simulink model "Transicao"  (R2015b)
settings: Solver=FixedStepAuto  StartTime=0  StopTime=120  FixedStep=sampleTime  RelTol=1e-3
InitFcn:
  | sampleTime = 0.01;
  | Ktd = 0.0526/1000;
  | Kdd = 0.0526/1000;
  | Lb = [0.27 0.27 0.27 0.27];
  | LbAssimetrico  = [0.27 0.27 0.18 0.36];
  | LbTeste  = [0.27 0.27 0.18 0.36];
  | Ixx = 0.0754483;
  | Iyy = 0.13642;
  | Izz = 0.2043333;
  | 
  | IXYZ = [Ixx 0 0; 0 Iyy 0; 0 0 Izz];
  | 
  | areaLateral = [0.0114398 0 0; 0 0.09533687 0; 0 0 0.33];
  | 
  | areaAsa = 0.243;
  | areaProfundor = 0.051;
  | densidadeAr = 1.2;
  | cdArrastoParasita = 1.5;
  | clAviao = 0.825;
  | cdAviao = 0.0743;
  | g = 9.8;
  | massa = 3;
  | velCruzeiro = 15;
  | 
  | inicioTransicao = 40;
  | inicioDesativaAtivacao = 80;
  | 
  | global kroll
  | global kpitch
  | global kyaw
  | 
  | global kx
  | global ky
  | global kz
  | 
  | %Voo em cruzeiro
  | global ku
  | global kzprof
  | global kpitchprof
undefined symbols (not defined in the file or in its folder): DiscIntNeverNeededParam, kpitch, kpitchprof, kroll, ku, kx, kyaw, kz, kzprof
libraries: simulink x17, aerolibwind2 x1
(part 2 of 2)

== matlab function Transicao/Dinâmica do sistema/Dinâmica do sistema ==
  data: w1 input; w2 input; w3 input; w4 input; estados output; gravidade input; massaTotal input; rho input; areaAviao input; areaAsa input; cdParasita input; cdAviao input; clAviao input; ktd input; kdd input; lb input; Ixyz input; velVento input; beta input; alphaProfundor input; dt input; estados_anterior input; U output; a_angular output; a output; XYZ output; XYZ_ponto output; XYZ_ponto_ponto output; phi_theta_psi output; phi_theta_psi_ponto output; thrustX output; arrastoParasita output; arrastoInduzido output; sustentacao output; arrastoTotal output; forcas output; gravidadeVec output
function [estados, U, a_angular, a, XYZ, XYZ_ponto,XYZ_ponto_ponto, phi_theta_psi, phi_theta_psi_ponto, thrustX, arrastoParasita, arrastoInduzido, sustentacao, arrastoTotal, forcas, gravidadeVec]  = fcn(w1,w2, w3, w4, gravidade, massaTotal,rho,areaAviao, areaAsa, cdParasita, cdAviao, clAviao, ktd, kdd, lb, Ixyz, velVento, beta, alphaProfundor, dt, estados_anterior)

XYZ = estados_anterior(:, 1);
XYZ_ponto = estados_anterior(:, 2);
phi_theta_psi = estados_anterior(:, 3);
phi_theta_psi_ponto = estados_anterior(:, 4);

roll = phi_theta_psi(1);
pitch = phi_theta_psi(2);
yaw = phi_theta_psi(3);

% for i = 1:numel(phi_theta_psi_ponto);
%    if(abs(phi_theta_psi_ponto(i)) < 10e-8)
%       phi_theta_psi_ponto(i) = 0;
%    end
%    
% end
% 
% % for i = 1:numel(theta_phi_psi);
% %    if(abs(theta_phi_psi(i)) < 10e-6)
% %       theta_phi_psi(i) = 0;
% %    end
% % end
% 
% for i = 1:numel(XYZ_ponto);
%    if(abs(XYZ_ponto(i)) < 10e-8)
%       XYZ_ponto(i) = 0;
%    end
% end

phi = roll;
theta = pitch;
psi = yaw;
% Matriz de rotação ZYX 
%matrizRotacao =     [cos(pitch)*cos(yaw) sin(roll)*sin(pitch)*cos(yaw)-cos(roll)*sin(yaw) cos(roll)*sin(pitch)*cos(yaw)+sin(roll)*sin(yaw);
%   cos(pitch)*sin(yaw) sin(roll)*sin(pitch)*sin(yaw)+cos(roll)*cos(yaw) cos(roll)*sin(pitch)*sin(yaw)-sin(roll)*cos(yaw);
%   -sin(pitch) sin(roll)*cos(pitch) cos(roll)*cos(pitch)];

%matrizRotacao =     [cos(phi)*cos(psi)-cos(theta)*sin(phi)*sin(psi) -cos(psi)*sin(phi)-cos(phi)*cos(theta)*sin(psi) sin(theta)*sin(psi) ;
%                     cos(theta)*cos(psi)*sin(phi)+cos(phi)*sin(psi) cos(phi)*cos(theta)*cos(psi)-sin(phi)*sin(psi) -cos(psi)*sin(theta) ;
%                     sin(phi)*sin(theta) cos(phi)*sin(theta) cos(theta)];

matrizRotacao =     [cos(theta)*cos(psi) cos(psi)*sin(theta)*sin(phi)-sin(psi)*cos(phi) cos(psi)*sin(theta)*cos(phi)+sin(psi)*sin(phi);
                     sin(psi)*cos(theta) sin(psi)*sin(theta)*sin(phi)+cos(psi)*cos(phi) sin(psi)*sin(theta)*cos(phi)-cos(psi)*sin(phi);
                     -sin(theta) cos(theta)*sin(phi) cos(theta)*cos(phi)];



%T = [1 sin(roll)*tan(pitch) cos(roll)*tan(pitch);
%    0 cos(roll) -sin(roll);
%    0 sin(roll)/cos(pitch) cos(roll)/cos(pitch)];

T = [1 0 -sin(theta);
    0 cos(phi) cos(theta)*sin(phi);
    0 -sin(phi) cos(theta)*cos(phi)];

% Encontra velocidades lineares e angulares no eixo do corpo com base no
% eixo inercial
vel_angular_body = T*phi_theta_psi_ponto;
vel_linear_body = matrizRotacao'*XYZ_ponto;

%Velocidade do vento no referencial do corpo
vel_vento_body = matrizRotacao'*velVento;

% Velocidade do corpo em relação ao vento
vel_aerodinamica_body = vel_linear_body-vel_vento_body;

w2ParaU = [ ktd      ktd     ktd      ktd;
           -ktd*lb(2)      ktd*lb(1)     ktd*lb(1)     -ktd*lb(2);
            ktd*lb(3)     -ktd*lb(4)     ktd*lb(3)     -ktd*lb(4);
           -kdd     -kdd       kdd      kdd];


       
U = w2ParaU * [w1^2*cos(beta); w2^2; w3^2*cos(beta); w4^2]; % Componente vertical, motor 1 e 3 estão em tilt com ângulo Beta
thrustX = [([ ktd      ktd     ktd      ktd]*[w1^2*sin(beta); 0; w3^2*sin(beta); 0]) ; 0 ; 0];% Componente da força horizontal, com motor tiltado

% Forças presentes no body frame axis
thrust = U(1)*[0; 0; 1];
forcas = -thrust;
arrastoParasita = -sign(vel_aerodinamica_body).*((rho*(vel_aerodinamica_body.^2)'*cdParasita*areaAviao/2)'); % Calcula arrasto parasita

if(vel_aerodinamica_body(1) > 0)
    arrastoInduzido = [-rho*vel_aerodinamica_body(1)^2*cdAviao*areaAsa/2 ; 0 ; 0]; % Encontra arrasto induzido da asa + profundor (o cd ta ajustado pra usar apenas a área da asa)
    clAlpha = 0.0744*(theta*180/pi +6) + 0.148;
    sustentacao = [0 ; 0 ; -rho*vel_aerodinamica_body(1)^2*clAlpha*areaAsa/2];
else
     arrastoInduzido = [0;0;0];
     sustentacao = [0;0;0];
end
arrastoTotal = arrastoParasita+arrastoInduzido;
gravidadeVec = (matrizRotacao')*(massaTotal*gravidade*[0; 0; 1]);
FtotalBody = -thrust + gravidadeVec + arrastoParasita+arrastoInduzido+sustentacao + thrustX; 

% Momentos presentes no body frame axis
mXroll = U(2);
mYpitch = U(3)+alphaProfundor;
mZyaw = U(4);
momentos = [mXroll; mYpitch; mZyaw];

% Adiciona efeito giroscópio e efeitos do produto vetorial do modelo de
% Newton-Euler
FtotalBody = FtotalBody - cross(vel_angular_body,(massaTotal*vel_linear_body));
momentos = momentos - cross(vel_angular_body,(Ixyz*vel_angular_body));

% Calcula aceleração em relação ao body frame
a = FtotalBody/massaTotal;

%Calcula aceleração angular em relação ao body frame
a_angular = inv(Ixyz)*(momentos);
%a_angular = inv(Ixyz)*(momentos);

% Resolvendo as tretas dos ângulos 
% https://i.imgur.com/82268P1.png
% Fonte: modelagem tese irada maluca

% Calcula velocidade angular em relação ao body axis
vel_angular_body = vel_angular_body + a_angular*dt;

% Encontra velocidade angular em relação ao eixo inercial
phi_theta_psi_ponto = inv(T)*vel_angular_body;

% Encontra os ângulos com base na velocidade angular no eixo inercial
phi_theta_psi = phi_theta_psi+ phi_theta_psi_ponto*dt;

% Encontra velocidade linear em relação ao body axis
vel_linear_body = vel_linear_body + a*dt;

XYZ_ponto_ponto = matrizRotacao*a;

% Encontra velocidade linear em relação ao eixo inercial
XYZ_ponto = matrizRotacao*vel_linear_body;

% Encontra posição em relação ao eixo inercial
XYZ = XYZ+XYZ_ponto*dt;

% if(modoCruzeiro == 1)
%     phi_theta_psi(2) = 0;
%     phi_theta_psi_ponto(2) = 0;
% end

estados = horzcat(XYZ, XYZ_ponto, phi_theta_psi, phi_theta_psi_ponto);

== matlab function Transicao/Atuador VTOL/Motor mixer ==
  data: u1thrust input; w1 output; u2mRoll input; u3mPitch input; u4mYaw input; w2 output; w3 output; w4 output; ktd input; kdd input; lb input
% Transforma um comando de thrust e momento em velocidade angular
function [w1,w2,w3,w4]= fcn(u1thrust, u2mRoll, u3mPitch, u4mYaw, ktd, kdd, lb)
% Supondo que U seja força e momentos
%w2ParaU = [ Ktd      Ktd     Ktd      Ktd;
%          -Ktd*Lb   Ktd*Lb  Ktd*Lb  -Ktd*Lb;
%           Ktd*Lb  -Ktd*Lb  Ktd*Lb  -Ktd*Lb;
%          -Kdd     -Kdd     Kdd      Kdd]

w2ParaU = [ ktd      ktd     ktd      ktd;
           -ktd*lb(2)      ktd*lb(1)     ktd*lb(1)     -ktd*lb(2);
            ktd*lb(3)     -ktd*lb(4)     ktd*lb(3)     -ktd*lb(4);
           -kdd     -kdd       kdd      kdd];


w = inv(w2ParaU)*[u1thrust ; u2mRoll ; u3mPitch ; u4mYaw];
for i = 1:numel(w);
   if(w(i) > 837.75^2)
      w(i) = 837.75^2; 
   end
end
for i = 1:numel(w);
   if(w(i) < 0)
      w(i) = 0; 
   end
end

w1 = sqrt(w(1));
w2 = sqrt(w(2));
w3 = sqrt(w(3));
w4 = sqrt(w(4));

== matlab function Transicao/Controle ângulo tilt/Controle Gain Schedualing ==
  data: velocidadeInercial input; phi_theta_psi input; betaFixo input; velAngularBeta input; tempoAtivacao input; sampleTime input; tempoSim input; betaAnterior input; beta output; velCruzeiro input; velCorpo output; modoAsaAnterior input; tempoDesativacao input
function [beta, velCorpo] = fcn(velocidadeInercial, phi_theta_psi, betaFixo, velAngularBeta, tempoAtivacao, sampleTime, tempoSim, betaAnterior, velCruzeiro, modoAsaAnterior, tempoDesativacao)
% Transforma um comando de thrust e momento em velocidade angular
velCorpo = [0;0;0];
beta = betaAnterior;
roll = phi_theta_psi(1);
pitch = phi_theta_psi(2);
yaw = phi_theta_psi(3);

phi = roll;
theta = pitch;
psi = yaw;

matrizRotacao =     [cos(theta)*cos(psi) cos(psi)*sin(theta)*sin(phi)-sin(psi)*cos(phi) cos(psi)*sin(theta)*cos(phi)+sin(psi)*sin(phi);
                     sin(psi)*cos(theta) sin(psi)*sin(theta)*sin(phi)+cos(psi)*cos(phi) sin(psi)*sin(theta)*cos(phi)-cos(psi)*sin(phi);
                     -sin(theta) cos(theta)*sin(phi) cos(theta)*cos(phi)];
                 
velCorpo = matrizRotacao'*velocidadeInercial;

if(tempoSim >= tempoAtivacao)
   if(betaAnterior < pi/2)
       beta = betaAnterior + velAngularBeta*sampleTime;
   end
   if(betaAnterior >= betaFixo)
       beta = betaFixo;
   end
else
   beta = 0; 
end

if(tempoSim >= tempoDesativacao)
    if(beta >=0)
       beta = betaAnterior - velAngularBeta*sampleTime;
    else
       beta =0;
    end
end

% if(beta < pi/6)
%    beta até pi/6
%     xPitchX = [3.3677    0.4996    0.0200    0.2366    1.9994    0.5776    0.9994    0.0200]
%     xZ = [1.0370    7.9791    1.4905    0.0191    1.2406]
%     display('parou aqui')
% else
%     xPitchX = [7.1864    4.9121    0.1706    1.1068   1.9994    0.5776    0.9994    0.0200]
%     xZ = [0.1    20    2.5    0    0.5]
% end
% 
% kpitch.kp = xPitchX(1);
% kpitch.kp_ponto = xPitchX(2);
% kpitch.kd_ponto = xPitchX(3);
% kpitch.ki_ponto = xPitchX(4);
% kz.kp = xZ(1);
% kz.kp_ponto = xZ(2);
% kz.kp_ponto_ponto = xZ(3);
% kz.kd_ponto_ponto = xZ(4);
% kz.ki_ponto_ponto = xZ(5);


% if(modoAsaAnterior == 1)
%         if(tempoSim >= tempoDesativacao)
%             if(beta >=0)
%                beta = betaAnterior - velAngularBeta*sampleTime;
%                modoAsa = 0;
%             else
%                beta =0;
%             end
%         end
% end
% 
% if(modoAsa == 1)
%     phi_theta_psi_profundor(2) = phi_theta_psi(2)/(((tempoSim-tempoAtivacao)+1)^2)
% end

== matlab function Transicao/Interface gráfica1/Desenho do drone ==
  data: desenhoDrone output
function desenhoDrone = fcn

%Retângulo com o espaçamento dos motores
%Braço Motor 1
p1 = [-0.54 -0.54 0];
p2 = [0.54 -0.54 0];
%Braço Motor 2
p3 = [0.54 0.54 0];
p4 = [-0.54 0.54 0]; 
%Braço quad
p5 = [0 -1 0];
p6 = [0 1 0];

%boom
p7 = [0 0 0];
p8 = [-1 0 0];

%profundor
p9 = [-1 -0.3 0];
p10 = [-1 0.3 0];

%leme
p11 = [-1 0 0];
p12 = [-1 0 0.3];

desenhoDrone = [[p1(1) p2(1) p3(1) p4(1) p5(1) p6(1) p7(1) p8(1) p9(1) p10(1) p11(1) p12(1)]; [p1(2) p2(2) p3(2) p4(2) p5(2) p6(2) p7(2) p8(2) p9(2) p10(2) p11(2) p12(2)]; [p1(3) p2(3) p3(3) p4(3) p5(3) p6(3) p7(3) p8(3) p9(3) p10(3) p11(3) p12(3)]];

== matlab function Transicao/Interface gráfica1/Rotacao ==
  data: vetorNoEixoDoCorpo input; vetorNoEixoInercial output; PitchRollYaw input; XYZ input
function vetorNoEixoInercial = fcn(vetorNoEixoDoCorpo, PitchRollYaw, XYZ)
pitch = PitchRollYaw(1);
roll = PitchRollYaw(2);
yaw = PitchRollYaw(3);


matrizRotacao =     [cos(pitch)*cos(yaw) sin(roll)*sin(pitch)*cos(yaw)-cos(roll)*sin(yaw) cos(roll)*sin(pitch)*cos(yaw)+sin(roll)*sin(yaw);
   cos(pitch)*sin(yaw) sin(roll)*sin(pitch)*sin(yaw)+cos(roll)*cos(yaw) cos(roll)*sin(pitch)*sin(yaw)-sin(roll)*cos(yaw);
   -sin(pitch) sin(roll)*cos(pitch) cos(roll)*cos(pitch)];

% matrizRotacao =     [cos(pitch)*cos(yaw) sin(roll)*sin(pitch)*cos(yaw)-cos(roll)*sin(yaw) cos(roll)*sin(pitch)*cos(yaw)+sin(roll)*sin(yaw);
%     cos(pitch)*sin(yaw) sin(roll)*sin(pitch)*sin(yaw)+cos(roll)*cos(yaw) cos(roll)*sin(pitch)*sin(yaw)-sin(roll)*cos(yaw);
%     -sin(pitch) sin(roll)*cos(pitch) cos(roll)*cos(pitch)]

vetorNoEixoInercial = matrizRotacao*vetorNoEixoDoCorpo;
vetorNoEixoInercial = vetorNoEixoInercial + repmat(XYZ,1,size(vetorNoEixoInercial, 2));

== matlab function Transicao/Controle ângulo tilt/Controle Gain Schedualing1 ==
  data: velocidadeInercial input; phi_theta_psi input; betaFixo input; velAngularBeta input; tempoAtivacao input; sampleTime input; tempoSim input; betaAnterior input; beta output; velCruzeiro input; velCorpo output; modoAsaAnterior input; tempoDesativacao input
% Transforma um comando de thrust e momento em velocidade angular
function [beta, velCorpo] = fcn(velocidadeInercial, phi_theta_psi, betaFixo, velAngularBeta, tempoAtivacao, sampleTime, tempoSim, betaAnterior, velCruzeiro, modoAsaAnterior, tempoDesativacao)
modoAsa = modoAsaAnterior;
velCorpo = [0;0;0];
beta = betaAnterior;
roll = phi_theta_psi(1);
pitch = phi_theta_psi(2);
yaw = phi_theta_psi(3);

phi = roll;
theta = pitch;
psi = yaw;

matrizRotacao =     [cos(theta)*cos(psi) cos(psi)*sin(theta)*sin(phi)-sin(psi)*cos(phi) cos(psi)*sin(theta)*cos(phi)+sin(psi)*sin(phi);
                     sin(psi)*cos(theta) sin(psi)*sin(theta)*sin(phi)+cos(psi)*cos(phi) sin(psi)*sin(theta)*cos(phi)-cos(psi)*sin(phi);
                     -sin(theta) cos(theta)*sin(phi) cos(theta)*cos(phi)];
                 
velCorpo = matrizRotacao'*velocidadeInercial;

if(modoAsaAnterior == 0)
    if(tempoSim >= tempoAtivacao)
       if((velCorpo(1) <= velCruzeiro) && (betaAnterior < betaFixo))
           beta = betaAnterior + velAngularBeta*sampleTime;
           modoAsa = 0;
       end
       if((velCorpo(1) <= velCruzeiro) && (betaAnterior >= betaFixo) )
           beta = betaAnterior; 
           modoAsa = 0;
       end
       if((velCorpo(1) > velCruzeiro) && betaAnterior < pi/2)
           beta = betaAnterior + velAngularBeta*sampleTime;
           modoAsa = 0;
       end
       if((velCorpo(1) > velCruzeiro) && betaAnterior >= pi/2)
           beta = pi/2;
           modoAsa = 1;
       end
    else
       beta = 0; 
    end
end


if(modoAsaAnterior == 1)
        if(tempoSim >= tempoDesativacao)
            if(beta >=0)
               beta = betaAnterior - velAngularBeta*sampleTime;
               modoAsa = 0;
            else
               beta =0;
            end
        end
end
% 
% if(modoAsa == 1)
%     phi_theta_psi_profundor(2) = phi_theta_psi(2)/(((tempoSim-tempoAtivacao)+1)^2)
% end

== matlab function Transicao/Interface gráfica1/desenhaVetores ==
  data: vetorNoEixoDoCorpo input; vetorNoEixoInercial input
function fcn(vetorNoEixoDoCorpo, vetorNoEixoInercial)
coder.extrinsic('quiver3');

coder.extrinsic('fill3');
%Desenha eixo Inercial
quiver3(0,0,0, 1, 0, 0);
hold on
quiver3(0,0,0, 0, 1, 0);
quiver3(0,0,0, 0, 0, 1);
vetorNoEixoInercial(1, :);

plot3(vetorNoEixoInercial(1, 1:2), vetorNoEixoInercial(2, 1:2), vetorNoEixoInercial(3, 1:2), 'LineWidth', 2, 'LineJoin', 'round');
plot3(vetorNoEixoInercial(1, 3:4), vetorNoEixoInercial(2, 3:4), vetorNoEixoInercial(3, 3:4), 'LineWidth', 2, 'LineJoin', 'round');
plot3(vetorNoEixoInercial(1, 5:6), vetorNoEixoInercial(2, 5:6), vetorNoEixoInercial(3, 5:6), 'LineWidth', 6, 'LineJoin', 'round');
plot3(vetorNoEixoInercial(1, 7:8), vetorNoEixoInercial(2, 7:8), vetorNoEixoInercial(3, 7:8), 'LineWidth', 3, 'LineJoin', 'round');
plot3(vetorNoEixoInercial(1, 9:10), vetorNoEixoInercial(2, 9:10), vetorNoEixoInercial(3, 9:10), 'LineWidth', 3, 'LineJoin', 'round');
plot3(vetorNoEixoInercial(1, 11:12), vetorNoEixoInercial(2, 11:12), vetorNoEixoInercial(3, 11:12), 'LineWidth', 3, 'LineJoin', 'round');
xlabel('x'); ylabel('y'); zlabel('z');  

axis([-10 10 -10 10 -1 10]);
hold off
